simulink model "UNO_Servo_task"  (Simulink 3.00)
libraries: REXduino_library x4, mathlib x4, genlib x2

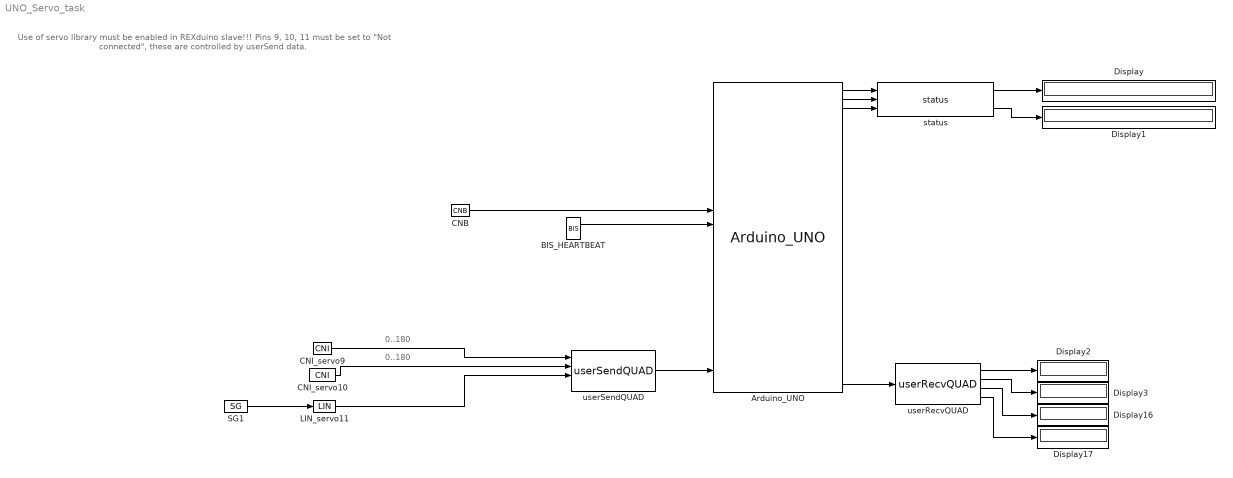
== system UNO_Servo_task ==
  note: 0..180
  note: 0..180
  note: Use of servo library must be enabled in REXduino slave!!!
      |
      | Pins 9, 10, 11 must be set to "Not connected", these are controlled by userSend data.
  Arduino_UNO : REXduino_library/Arduino_UNO  comPort=/dev/ttyACM0  pinmode2=1: Not connected  pinmode3=1: Not connected  pinmode4=1: Not connected  pinmode5=1: Not connected  pinmode6=1: Not connected  pinmode9=1: Not connected  pinmode10=1: Not connected  pinmode11=1: Not connected  pinmodeA0=1: Not connected  pinmodeA1=1: Not connected  pinmodeA2=1: Not connected  pinmodeA3=1: Not connected  pinmodeA4=1: Not connected  pinmodeA5=1: Not connected  usercmd=2: Four bytes
  BIS_HEARTBEAT : genlib/BIS  Y0=off  t1=0.7  t2=0.8  t3=0.9  t4=1.0  t5=0  t6=6  t7=7  t8=8  RPT=on  bEdit=off
  CNB : mathlib/CNB  YCN=on
  CNI_servo10 : mathlib/CNI  icn=111
  CNI_servo9 : mathlib/CNI  icn=90
  Display{,1..3,16..17} (6 alike) : Display
      settings: Format=Best fit
  LIN_servo11 : mathlib/LIN  u1=-1  y1=0  u2=1  y2=180
  SG1 : genlib/SG  isig=3: SAWTOOTH  amp=1  freq=0.1  phase=0  offset=0  ifrunit=1: Hz  iphunit=1: degrees
  status : REXduino_library/status
      mask Type: REX sequence
  userRecvQUAD : REXduino_library/userRecvQUAD
      mask Type: REX sequence
  userSendQUAD : REXduino_library/userSendQUAD
      mask Type: REX sequence
  wires:
  Arduino_UNO/1 -> status/1
  Arduino_UNO/2 -> status/2
  Arduino_UNO/3 -> status/3
  Arduino_UNO/34 -> userRecvQUAD/1
  BIS_HEARTBEAT/1 -> Arduino_UNO/10
  CNB/1 -> Arduino_UNO/9
  CNI_servo10/1 -> userSendQUAD/2
  CNI_servo9/1 -> userSendQUAD/1
  LIN_servo11/1 -> userSendQUAD/3
  SG1/1 -> LIN_servo11/1
  status/1 -> Display/1
  status/2 -> Display1/1
  userRecvQUAD/1 -> Display2/1
  userRecvQUAD/2 -> Display3/1
  userRecvQUAD/3 -> Display16/1
  userRecvQUAD/4 -> Display17/1
  userSendQUAD/1 -> Arduino_UNO/21
